simulink model "audiometric_test 2"  (R2017b)
settings: Solver=VariableStepAuto  StartTime=0.0  StopTime=10.0  RelTol=1e-3
libraries: simulink x2, dspsnks4 x1
settings Model: Creator=fpier  LastModifiedBy=fpier

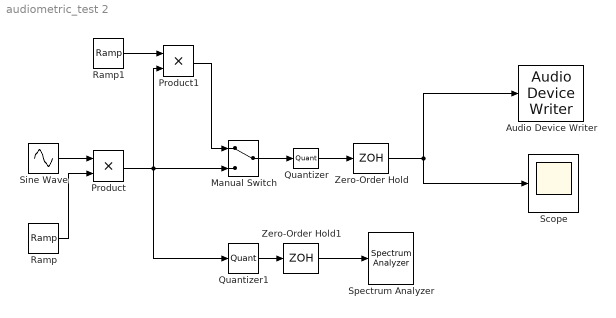
== system audiometric_test 2 ==
  Audio Device Writer : dspsnks4/Audio Device Writer  Driver=DirectSound  Device=Default  InheritSampleRate=on  SampleRate=44100  BitDepth=16-bit integer  BufferSize=4096  NumBuffers=10  DefaultOutputChannelMapping=on  OutputChannelMapping=1:2  OutputNumUnderrunSamples=off  DriverIdx=1  DeviceWarnFlag=''
  Manual Switch : ManualSwitch
  Product : Product
  Product1 : Product
  Quantizer : Quantizer  QuantizationInterval=0.0001
  Quantizer1 : Quantizer  QuantizationInterval=0.0001
  Ramp : simulink/Sources/Ramp  slope=2.5  start=0  X0=0
  Ramp1 : simulink/Sources/Ramp  slope=0.00001  start=0  X0=0
  Scope : Scope
  Sine Wave : Sin  Amplitude=0.0002  Frequency=2*pi*8000  SampleTime=1/44100
  Spectrum Analyzer : SpectrumAnalyzer
  Zero-Order Hold : ZeroOrderHold  SampleTime=-1
  Zero-Order Hold1 : ZeroOrderHold  SampleTime=-1
  wires:
  Quantizer/1 -> Zero-Order Hold/1
  Zero-Order Hold/1 -> Scope/1, Audio Device Writer/1
  Product/1 -> Product1/2, Quantizer1/1, Manual Switch/2
  Manual Switch/1 -> Quantizer/1
  Sine Wave/1 -> Product/1
  Ramp/1 -> Product/2
  Quantizer1/1 -> Zero-Order Hold1/1
  Zero-Order Hold1/1 -> Spectrum Analyzer/1
  Ramp1/1 -> Product1/1
  Product1/1 -> Manual Switch/1
